simulink model "part_two"  (R2019b)
settings: Solver=VariableStepAuto  StartTime=0.0  StopTime=100  RelTol=1e-3
values from neighbouring files (symbols this model uses):
  func_one = tf([-3 8.4 1.8], [1 13 32 20])    [part_two_params.m]
  func_two = tf([3], [1 6.3 11.8 8.7 9])    [part_two_params.m]
settings Model: Creator=adityaaaap  LastModifiedBy=adityaaaap
settings DataIOCC: ReturnWorkspaceOutputs=off
settings DebuggingCC: ArithmeticOperatorsInVariantConditions=warning
settings SFSimCC: SimUseLocalCustomCode=off  CustomCodeUndefinedFunction=UseInterfaceOnly
settings RTWCC: RTWUseLocalCustomCode=off
settings CodeAppCC: StateflowObjectComments=on

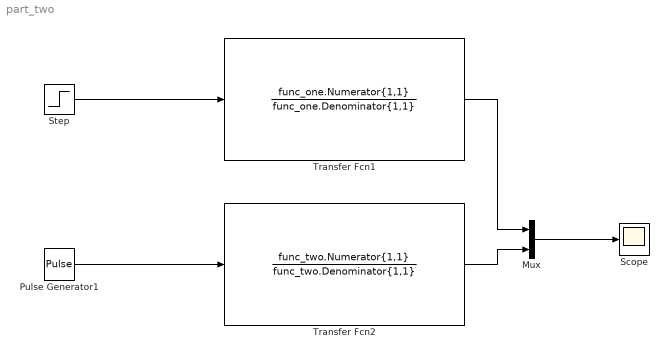
== system part_two ==
  Mux : Mux  Inputs=2
  Pulse Generator1 : DiscretePulseGenerator  Amplitude=0.5  Period=20  PulseWidth=5  SampleTime=0.001
  Scope : Scope
  Step : Step  Time=0  SampleTime=0.001
  Transfer Fcn1 : TransferFcn  Numerator=func_one.Numerator{1,1}  Denominator=func_one.Denominator{1,1}
  "Transfer Fcn2 " : TransferFcn  Numerator=func_two.Numerator{1,1}  Denominator=func_two.Denominator{1,1}
  wires:
  Step/1 -> Transfer Fcn1/1
  Transfer Fcn1/1 -> Mux/1
  "Transfer Fcn2 "/1 -> Mux/2
  Mux/1 -> Scope/1
  Pulse Generator1/1 -> "Transfer Fcn2 "/1
